simulink model "MotorPosCntrl"  (Simulink 8.6)
settings: Solver=ode45  StartTime=0.0  RelTol=1e-6
values from neighbouring files (symbols this model uses):
  C = Cc    [mem458Lab4CntrlDesign.m]
  D = Dc    [mem458Lab4CntrlDesign.m]
  K = 1    [mem458Lab4CntrlDesign.m]
  ref_position = 180    [mem458Lab4CntrlDesign.m]
  Ts = 0.01    [mem458Lab4CntrlDesign.m]
undefined symbols (not defined in the file or in its folder): A, B
settings Model: Creator=bcc88  LastModifiedBy=bcc88
settings OptimizationCC: BooleanDataType=off  ExpressionDepthLimit=128
settings DebuggingCC: SaveWithParameterizedLinksMsg=none  SignalResolutionControl=TryResolveAllWithWarning  SolverPrmCheckMsg=none  MultiTaskDSMMsg=warning  MultiTaskCondExecSysMsg=none  FcnCallInpInsideContextMsg=EnableAllAsError  StateNameClashWarn=none
settings HardwareCC: ProdBitPerPointer=64  ProdLargestAtomicFloat=Float  ProdIntDivRoundTo=Zero  ProdEndianess=LittleEndian  ProdWordSize=64  ProdHWDeviceType=Intel->x86-64 (Windows64)  TargetUnknown=on
settings GRTTargetCC: GeneratePreprocessorConditionals=Use local settings

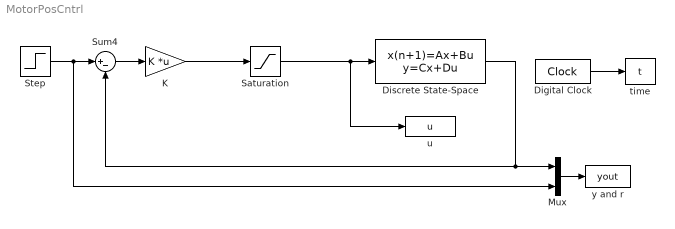
== system MotorPosCntrl ==
  Digital Clock : DigitalClock  SampleTime=Ts
  Discrete State-Space : DiscreteStateSpace  A=A  B=B  C=C  D=D  SampleTime=Ts
  K : Gain  Gain=K  Multiplication=Matrix(K*u)  SaturateOnIntegerOverflow=on  OutDataTypeStr=Inherit: Same as input  ParamDataTypeStr=Inherit: Same as input
  Mux : Mux  Inputs=2
  Saturation : Saturate  UpperLimit=100  LowerLimit=-100
  Step : Step  Time=0  After=ref_position  SampleTime=Ts
  Sum4 : Sum  Inputs=|+-  SaturateOnIntegerOverflow=on  InputSameDT=on  OutDataTypeStr=Inherit: Same as first input
  time : ToWorkspace  VariableName=t  SampleTime=-1
  u : ToWorkspace  VariableName=u  SampleTime=-1
  y and r : ToWorkspace  VariableName=yout  SampleTime=-1
  wires:
  Step/1 -> Sum4/1, Mux/2
  Digital Clock/1 -> time/1
  Mux/1 -> y and r/1
  Sum4/1 -> K/1
  Discrete State-Space/1 -> Mux/1, Sum4/2
  Saturation/1 -> u/1, Discrete State-Space/1
  K/1 -> Saturation/1
